simulink model "SimulinkProject"  (R2025b)
settings: Solver=ode5  StartTime=0.0  StopTime=60*5  FixedStep=1/16000  RelTol=1e-3
model workspace (MAT data in the model file):
  mass = 7
  radius = 333
undefined symbols (not defined in the file): DiscIntNeverNeededParam
libraries: simulink x5, simulink_extras x4, eeGeneralControl x2
settings Model: Creator=Fabian  LastModifiedBy=Fabian

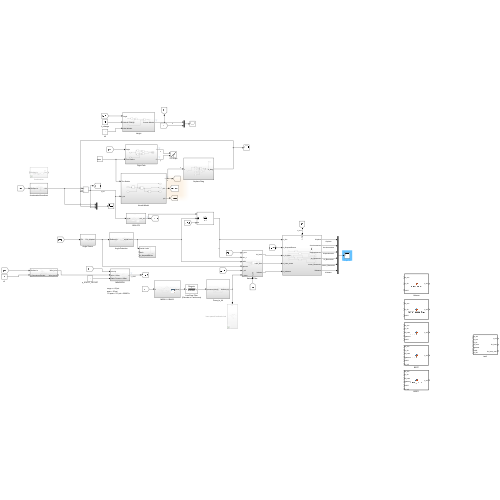
[thumbnail: Simulink's stored preview of the top-level diagram]
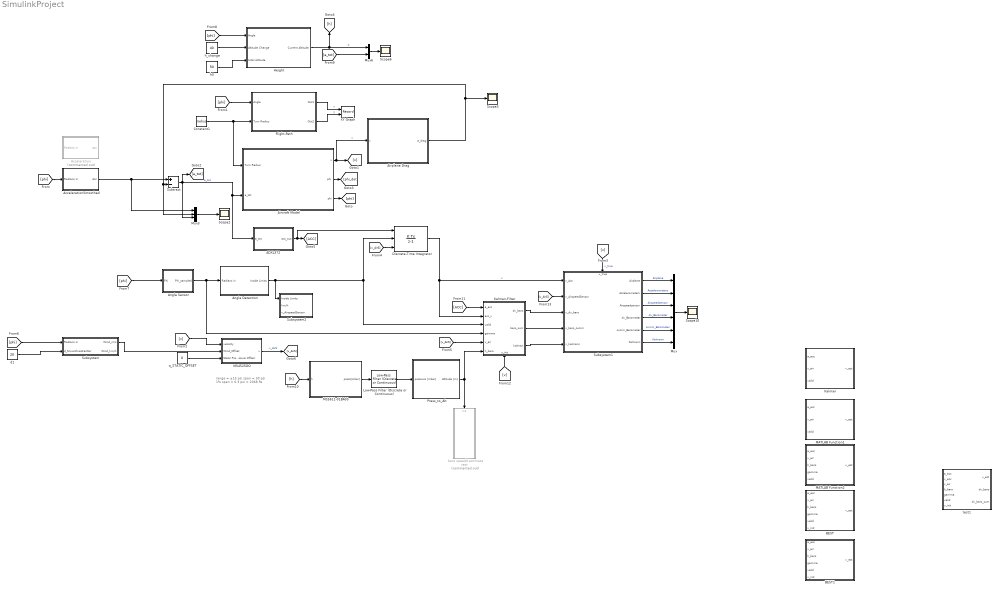
== system SimulinkProject ==
  note: range = ±15 psi
      | span = 30 psi
      | 1% span = 0.3 psi ≈ 2068 Pa
  ADXL372 : Subsystem
  Acceleration : Subsystem  Commented=on
  AccelerationSmoothed : Subsystem
  Aircraft Model : Subsystem
  Airplane Drag : Subsystem
  Angle Detection : Subsystem
  Angle Sensor : Subsystem
  BEST : MATLAB Function  TreatAsAtomicUnit=on
  BEST1 : MATLAB Function  TreatAsAtomicUnit=on
  Constant1 : Constant  Value=radius
  Discrete-Time Integrator : DiscreteIntegrator  ExternalReset=level  InitialConditionSource=external  SampleTime=1/3200  ICPrevOutput=DiscIntNeverNeededParam  ICPrevScaledInput=DiscIntNeverNeededParam
  Flight-Path : Subsystem
  Height : Subsystem
  Kalman : MATLAB Function  TreatAsAtomicUnit=on
  Kalman-Filter : Subsystem
      settings: PortSchema="{\"entries\":[{\"content\":{\"sides\":[{\"content\":{\"connectorIds\":[\"In1\",\"In2\",\"In3\",\"In4\",\"In5\",\"In6\"]},\"type\":\"ConnectorPlacement.EquallySpacedRectSide\",\"uuid\":\"52a043f1-34d7-4573-920f-90bbef37c175\"},{\"content\":{\"connectorIds\":[\"Out1\",\"Out2\",\"Out3\"],\"side\":\"RIGHT\"},\"type\":\"ConnectorPlacement.EquallySpacedRectSide\",\"uuid\":\"45beeb02-59fe-4ad5-aebe-ddb1f1721e27\"},{\"content\":{\"side\":\"TOP\"},\"type\":\"ConnectorPlacement.EquallySpacedRectSide\",\"uuid\":\"02723afe-8ee2-4376-9f83-f239e2e6ab52\"},{\"content\":{\"connectorIds\":[\"In7\"],\"side\":\"BOTTOM\"},\"type\":\"ConnectorPlacement.EquallySpacedRectSide\",\"uuid\":\"f847a05c-6e0c-45de-94de-b2ed33ea680b\"}]},\"type\":\"ConnectorPlacement.EquallySpacedConnector\",\"uuid\":\"0a8bc44f-e3ea-43fc-9907-5bdc9879c4d9\"}],\"packageUris\":[\"http://schema.mathworks.com/mf0/Connector/R2020b\"],\"version\":\"1.0\"}"
  Low-Pass Filter (Discrete or Continuous) : eeGeneralControl/Low-Pass Filter (Discrete or Continuous)  K=1  T=0.021  B=inf  A=-inf  init_option=Inherited from block input  x0=0  Ts=-1
  MATLAB Function1 : MATLAB Function  TreatAsAtomicUnit=on
  MATLAB Function2 : MATLAB Function  TreatAsAtomicUnit=on
  MS4525DO : Subsystem
  "MS5611-01BA03 " : Subsystem
  Mux : Mux  Inputs=6
  Mux3 : Mux  Inputs=3
  Mux6 : Mux  Inputs=2
  Press_to_Alt : Subsystem
  Scope{2..3,6,10} (4 alike) : Scope
      Scope10 settings: ActiveDisplayYMinimum=748.19267918173944  ActiveDisplayYMaximum=894.80486408784191  DataLoggingVariableName=ScopeData11
      Scope2 settings: ActiveDisplayYMinimum=-39.208466924616559  ActiveDisplayYMaximum=63.33696033694325  DataLoggingVariableName=ScopeData3
      Scope3 settings: ActiveDisplayYMinimum=-3.5843354434410593  ActiveDisplayYMaximum=33.486381490969542  DataLoggingVariableName=ScopeData6
      Scope6 settings: ActiveDisplayYMinimum=-31.394100237137991  ActiveDisplayYMaximum=92.400581276019  DataLoggingVariableName=ScopeData13
  Subsystem : Subsystem
  Subsystem1 : Subsystem
      settings: PortSchema="{\"entries\":[{\"content\":{\"sides\":[{\"content\":{\"connectorIds\":[\"In1\",\"In2\",\"In3\",\"In4\",\"In5\"]},\"type\":\"ConnectorPlacement.EquallySpacedRectSide\",\"uuid\":\"1310de41-fa36-4b52-bea7-0cc5965a0e40\"},{\"content\":{\"connectorIds\":[\"Out1\",\"Out2\",\"Out3\",\"Out4\",\"Out5\",\"Out6\"],\"side\":\"RIGHT\"},\"type\":\"ConnectorPlacement.EquallySpacedRectSide\",\"uuid\":\"190a2e70-065a-4914-8f4e-4e8426a30cbe\"},{\"content\":{\"connectorIds\":[\"In6\"],\"side\":\"TOP\"},\"type\":\"ConnectorPlacement.EquallySpacedRectSide\",\"uuid\":\"6c2c139e-493e-4709-bc4f-803947cf8aa6\"}]},\"type\":\"ConnectorPlacement.EquallySpacedConnector\",\"uuid\":\"13196e14-1744-4a93-b58c-eb55a0754985\"}],\"packageUris\":[\"http://schema.mathworks.com/mf0/Connector/R2020b\"],\"version\":\"1.0\"}"
  Subsystem2 : Subsystem
  Subtract : Sum  Inputs=+-
  XY Graph : Record  NumPorts=2.0  FileSettingsInternal="{\"entries\":[{\"content\":{\"excelSettings\":{\"content\":{},\"type\":\"Streamout.ExcelSettings\"},\"parquetSettings\":{\"content\":{},\"type\":\"Streamout.ParquetSettings\"}},\"type\":\"Streamout.FileSettingStorage\",\"uuid\":\"\"}],\"packageUris\":[\"http:\\/\\/schema.mathworks.com\\/mf0\\/streamout_blocks\\/R2020a\"],\"version\":\"1.0\"}"  FrameSettings=[0, 0]  Layout=[1 1]  SignalsInternal="{\"entries\":[{\"content\":{\"signals\":[{\"content\":{\"blockPath\":[],\"dimensions\":[1],\"domain\":\"\",\"lineColor\":\"#a2142f\",\"plots\":[ 1 ],\"port\":1,\"sid\":[\"\"],\"signalID\":1,\"signalName\":\"x\"},\"type\":\"RecordBlkView.Signal\",\"uuid\":\"\"},{\"content\":{\"blockPath\":[],\"dimensions\":[1],\"domain\":\"\",\"lineColor\":\"#139fff\",\"plots\":[ 1 ],\"port\":2,\"sid\":[\"\"],\"signalID\":2,\"signalName\":\"y\"},\"type\":\"RecordBlkView.Signal\",\"uuid\":\"\"}]},\"type\":\"RecordBlkView.InputSignals\",\"uuid\":\"\"}],\"packageUris\":[\"http:\\/\\/schema.mathworks.com\\/mf0\\/streamout_blocks\\/R2020a\"],\"version\":\"1.0\"}"  VisualizationBindings="{\"xyplotplugin\":{\"info\":[{\"series\":[{\"bindingParametersList\":[{\"parameter\":\"X-Axis\",\"signalID\":1,\"signalName\":\"x\"},{\"parameter\":\"Y-Axis\",\"signalID\":2,\"signalName\":\"y\"}],\"seriesID\":0}],\"subplotID\":1}]}}"  CompatibilityTag=XY
  baro speedd estimate test : Subsystem  Commented=on
  d1 : Constant  Value=20
  h0 : Constant  Value=50
  h_change : Constant  Value=40
  q_STATIC_OFFSET : Constant  Value=0
  test1 : MATLAB Function  TreatAsAtomicUnit=on
  wires:
  Subtract/1 -> [a_tot], ADXL372/1(a_tot), Aircraft Model/2(a_tot), Mux3/3  "a_tot"
  Constant1/1 -> Flight-Path/2(Turn Radius), Aircraft Model/1(Turn Radius)
  [phi] -> AccelerationSmoothed/1(Radians in)
  [v] -> MS4525DO/1(velocity)
  q_STATIC_OFFSET/1 -> MS4525DO/3(Static Pressure Offset)
  [phi] -> Flight-Path/1(Angle)
  Flight-Path/1(Out1) -> XY Graph/1  "x"
  Flight-Path/2(Out2) -> XY Graph/2  "y"
  Aircraft Model/1(v) -> Airplane Drag/1(v), [v]  "v"
  Aircraft Model/2(phi.) -> [phi_dot]
  Aircraft Model/3(phi) -> [phi]
  Mux3/1 -> Scope2/1
  [phi] -> Subsystem/1(Radians in)
  d1/1 -> Subsystem/2(d_SmoothnesFacttor)
  Subsystem/1(Wind_m/s) -> MS4525DO/2(Wind_Offset)
  AccelerationSmoothed/1(Acc) -> Mux3/1, Subtract/1
  [phi] -> Angle Sensor/1(Phi)
  h0/1 -> Height/3(Inital altitude)
  h_change/1 -> Height/2(Altitude Change)
  [phi] -> Height/1(Angle)
  Mux6/1 -> Scope6/1
  Height/1(Current Altitude) -> [h], Mux6/1  "h"
  [a_tot] -> Mux6/2
  [h] -> "MS5611-01BA03 "/1(h)
  Airplane Drag/1(a_drag) -> Mux3/2, Subtract/2, Scope3/1
  Discrete-Time Integrator/1 -> Kalman-Filter/2(acc_v), Subsystem1/1(v_Acc)  "v"
  "MS5611-01BA03 "/1(press[mbar]) -> Low-Pass Filter (Discrete or Continuous)/1
  Press_to_Alt/1(Altitude [m]) -> Kalman-Filter/6(h_baro), baro speedd estimate test/1(In1)
  Low-Pass Filter (Discrete or Continuous)/1 -> Press_to_Alt/1(pressure [mbar])
  Angle Sensor/1(Phi_sampled) -> Kalman-Filter/4(gamma), Angle Detection/1(Radians in)
  Angle Detection/1(Inside Limits) -> Subsystem2/1(Inside Limits), Kalman-Filter/3(valid), Discrete-Time Integrator/2
  ADXL372/1(acc_out) -> Discrete-Time Integrator/1, [ACC]
  [ACC] -> Kalman-Filter/1(a_acc)
  [v] -> Kalman-Filter/7(v_init)
  MS4525DO/1(v) -> [v_AirS]  "v_AirS"
  [v_AirS] -> Discrete-Time Integrator/3
  [v_AirS] -> Kalman-Filter/5(v_air)
  [v] -> Subsystem1/6(v_true)  "v_true"
  [v_AirS] -> Subsystem1/2(v_AirspeedSensor)
  Kalman-Filter/1(dv_baro) -> Subsystem1/3(v_dv_baro)
  Kalman-Filter/2(baro_sum) -> Subsystem1/4(v_baro_summ)
  Kalman-Filter/3(kalman) -> Subsystem1/5(v_kalmann)
  Mux/1 -> Scope10/1
  Subsystem1/1(Airplane) -> Mux/1  "Airplane"
  Subsystem1/2(Accelerometers) -> Mux/2  "Accelerometers"
  Subsystem1/3(Airspeedsensor) -> Mux/3  "Airspeedsensor"
  Subsystem1/4(dv_Barometer) -> Mux/4  "dv_Barometer"
  Subsystem1/5(summ_Barometer) -> Mux/5  "summ_Barometer"
  Subsystem1/6(Kalmann) -> Mux/6  "Kalmann"

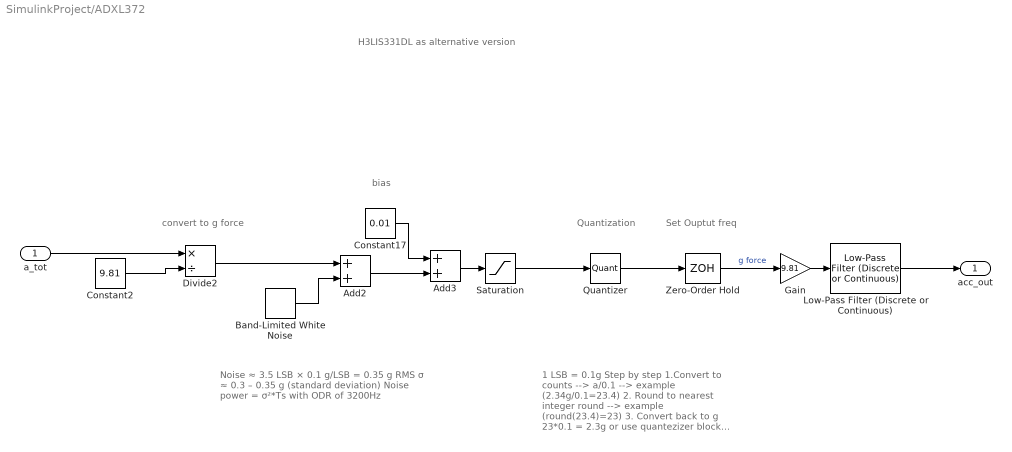
== system SimulinkProject/ADXL372 ==
  note: H3LIS331DL as alternative version
  note: convert to g force
  note: Noise ≈ 3.5 LSB × 0.1 g/LSB = 0.35 g RMS
      | σ ≈ 0.3 – 0.35 g (standard deviation)
      | Noise power = σ²*Ts
      | with ODR of 3200Hz
  note: bias
  note: Quantization
  note: 1 LSB = 0.1g
      | Step by step
      |
      | 1.Convert to counts
      | --> a/0.1 --> example (2.34g/0.1=23.4)
      | 2. Round to nearest integer
      | round --> example (round(23.4)=23)
      | 3. Convert back to g
      | 23*0.1 = 2.3g
      |
      | or use quantezizer block with 0.1
  note: Set Ouptut freq
  a_tot : Inport
  Add2 : Sum
  Add3 : Sum
  Band-Limited White Noise : simulink/Sources/Band-Limited White Noise  Cov=((0.35)^2)*(1/3200)  Ts=1/3200  seed=[23341]
  Constant17 : Constant  Value=0.01
  Constant2 : Constant  Value=9.81
  Divide2 : Product  Inputs=*/
  Gain : Gain  Gain=9.81
  Low-Pass Filter (Discrete or Continuous) : eeGeneralControl/Low-Pass Filter (Discrete or Continuous)  K=1  T=1/(2*pi*10)  B=inf  A=-inf  init_option=Inherited from block input  x0=0  Ts=1/3200
  Quantizer : Quantizer  QuantizationInterval=0.1
  Saturation : Saturate  UpperLimit=200  LowerLimit=-200
  Zero-Order Hold : ZeroOrderHold  SampleTime=1/3200
  acc_out : Outport
  wires:
  Constant2/1 -> Divide2/2
  Add3/1 -> Saturation/1
  Saturation/1 -> Quantizer/1
  Divide2/1 -> Add2/1
  Gain/1 -> Low-Pass Filter (Discrete or Continuous)/1
  Add2/1 -> Add3/2
  Constant17/1 -> Add3/1
  Band-Limited White Noise/1 -> Add2/2
  Quantizer/1 -> Zero-Order Hold/1
  Zero-Order Hold/1 -> Gain/1  "g force"
  Low-Pass Filter (Discrete or Continuous)/1 -> acc_out/1
  a_tot/1 -> Divide2/1

== system SimulinkProject/Acceleration ==
  note: Case 0 --> (0>value<120)
      | Case 1 --> (120>value<200)
      | Case 2 --> (200>value <360)
  Radians in : Inport
  1-D Lookup Table : Lookup_n-D  NumberOfTableDimensions=1  BreakpointsForDimension1=[0 120 130 190 210 360]  Table=[-3 -3 6 6 4 4]  InterpMethod=Linear Lagrange  InternalRulePriority=Speed  RndMeth=Simplest
  Constant4 : Constant  Value=360
  Math Function : Math  Operator=mod
  Radians to Degrees : simulink_extras/Transformations/Radians to Degrees
  Scope1 : Scope
      settings: ActiveDisplayYMinimum=2.9529948597935629  ActiveDisplayYMaximum=755.41634315848091
  Acc : Outport
  wires:
  Radians to Degrees/1 -> Math Function/1
  Constant4/1 -> Math Function/2
  Math Function/1 -> Scope1/1, 1-D Lookup Table/1
  Radians in/1 -> Radians to Degrees/1
  1-D Lookup Table/1 -> Acc/1

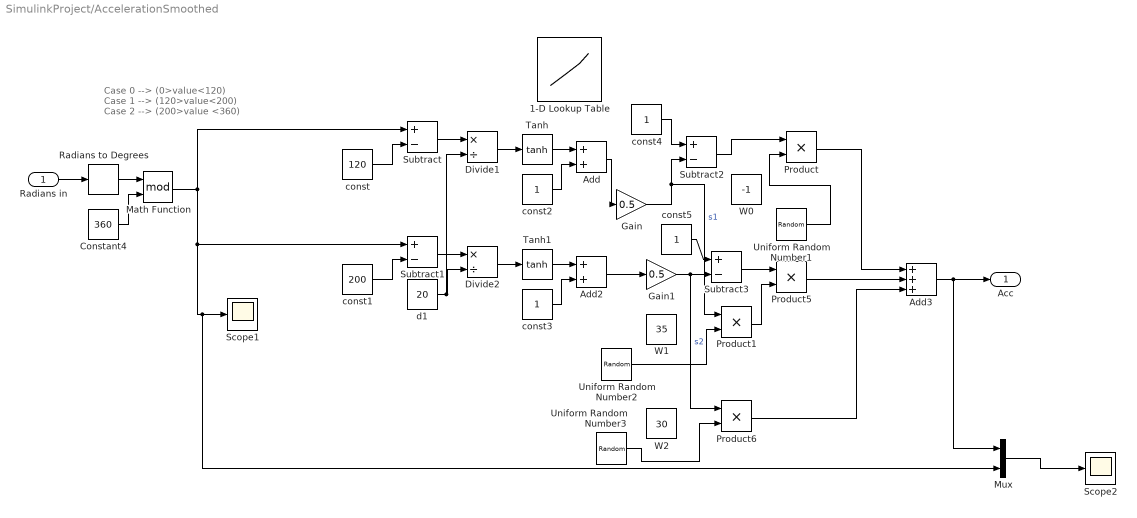
== system SimulinkProject/AccelerationSmoothed ==
  note: Case 0 --> (0>value<120)
      | Case 1 --> (120>value<200)
      | Case 2 --> (200>value <360)
  Radians in : Inport
  1-D Lookup Table : Lookup_n-D  NumberOfTableDimensions=1  BreakpointsForDimension1=[0 110 130 190 210 360]  Table=[-3 -3 6 6 4 4]  InterpMethod=Linear Lagrange  InternalRulePriority=Speed  RndMeth=Simplest
  Add : Sum
  Add2 : Sum
  Add3 : Sum  Inputs=+++
  Constant4 : Constant  Value=360
  Divide1 : Product  Inputs=*/
  Divide2 : Product  Inputs=*/
  Gain : Gain  Gain=0.5
  Gain1 : Gain  Gain=0.5
  Math Function : Math  Operator=mod
  Mux : Mux  Inputs=2
  Product{,1,5..6} (4 alike) : Product
  Radians to Degrees : simulink_extras/Transformations/Radians to Degrees
  Scope1 : Scope
      settings: ActiveDisplayYMinimum=-47.332509505790171  ActiveDisplayYMaximum=913.02258838484045
  Scope2 : Scope
      settings: ActiveDisplayYMinimum=-16.733117928341755  ActiveDisplayYMaximum=372.27391286785394  DataLoggingVariableName=ScopeData5
  Subtract{,1..3} (4 alike) : Sum  Inputs=+-
  Tanh : Trigonometry  Operator=tanh
  Tanh1 : Trigonometry  Operator=tanh
  Uniform Random Number1 : UniformRandomNumber  Minimum=-2  Maximum=0  SampleTime=0.1
  Uniform Random Number2 : UniformRandomNumber  Minimum=30  Maximum=40  SampleTime=0.1
  Uniform Random Number3 : UniformRandomNumber  Minimum=25  Maximum=35  SampleTime=0.1
  W0 : Constant  Value=-1
  W1 : Constant  Value=35
  W2 : Constant  Value=30
  const : Constant  Value=120
  const1 : Constant  Value=200
  const{2..5} (4 alike) : Constant
  d1 : Constant  Value=20
  Acc : Outport
  wires:
  Radians to Degrees/1 -> Math Function/1
  Constant4/1 -> Math Function/2
  Radians in/1 -> Radians to Degrees/1
  Math Function/1 -> Subtract1/1, Mux/2, Scope1/1, Subtract/1
  const4/1 -> Subtract2/1
  Tanh/1 -> Add/1
  const2/1 -> Add/2
  Add/1 -> Gain/1
  Product1/1 -> Product5/2
  Tanh1/1 -> Add2/1
  Subtract3/1 -> Product5/1
  Product6/1 -> Add3/3
  Subtract2/1 -> Product/1
  Subtract/1 -> Divide1/1
  const3/1 -> Add2/2
  Divide1/1 -> Tanh/1
  const/1 -> Subtract/2
  const1/1 -> Subtract1/2
  Subtract1/1 -> Divide2/1
  d1/1 -> Divide1/2, Divide2/2
  const5/1 -> Subtract3/1
  Gain1/1 -> Product6/1, Subtract3/2  "s2"
  Product5/1 -> Add3/2
  Add2/1 -> Gain1/1
  Gain/1 -> Subtract2/2, Product1/1  "s1"
  Divide2/1 -> Tanh1/1
  Product/1 -> Add3/1
  Add3/1 -> Mux/1, Acc/1
  Mux/1 -> Scope2/1
  Uniform Random Number1/1 -> Product/2
  Uniform Random Number2/1 -> Product1/2
  Uniform Random Number3/1 -> Product6/2

== system SimulinkProject/Aircraft Model ==
  Turn Radius : Inport
  a_tot : Inport  Port=2
  Divide1 : Product  Inputs=*/
  Integrator2 : Integrator  InitialCondition=13
  Integrator3 : Integrator  InitialCondition=pi
  v : Outport
  phi. : Outport  Port=2
  phi : Outport  Port=3
  wires:
  Divide1/1 -> phi./1, Integrator3/1  "phi."
  Integrator3/1 -> phi/1
  Integrator2/1 -> v/1, Divide1/1  "v"
  Turn Radius/1 -> Divide1/2
  a_tot/1 -> Integrator2/1

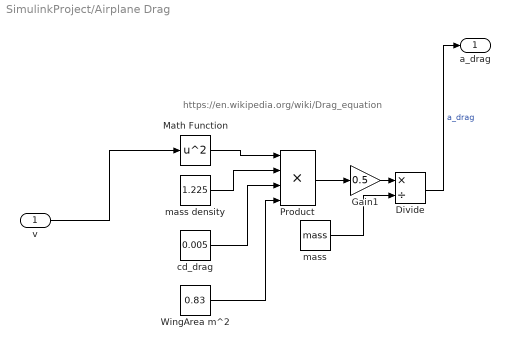
== system SimulinkProject/Airplane Drag ==
  note: https://en.wikipedia.org/wiki/Drag_equation
  v : Inport
  Divide : Product  Inputs=*/
  Gain1 : Gain  Gain=0.5
  Math Function : Math  Operator=square
  Product : Product  Inputs=4
  WingArea m^2 : Constant  Value=0.83
  cd_drag : Constant  Value=0.005
  mass : Constant  Value=mass
  mass density : Constant  Value=1.225
  a_drag : Outport
  wires:
  mass/1 -> Divide/2
  mass density/1 -> Product/2
  Divide/1 -> a_drag/1  "a_drag"
  Math Function/1 -> Product/1
  cd_drag/1 -> Product/3
  Gain1/1 -> Divide/1
  WingArea m^2/1 -> Product/4
  Product/1 -> Gain1/1
  v/1 -> Math Function/1

== system SimulinkProject/Angle Detection ==
  Radians in : Inport
  Compare To Constant : simulink/Logic and Bit Operations/Compare To Constant  relop=>=  const=50  OutDataTypeStr=boolean
  Compare To Constant1 : simulink/Logic and Bit Operations/Compare To Constant  relop=<=  const=80  OutDataTypeStr=boolean
  Constant4 : Constant  Value=360
  Logical Operator : Logic  AllPortsSameDT=off  OutDataTypeStr=fixdt(1,16)
  Math Function1 : Math  Operator=mod
  Radians to Degrees : simulink_extras/Transformations/Radians to Degrees
  Inside Limits : Outport
  wires:
  Math Function1/1 -> Compare To Constant/1, Compare To Constant1/1
  Compare To Constant/1 -> Logical Operator/1
  Compare To Constant1/1 -> Logical Operator/2
  Radians to Degrees/1 -> Math Function1/1
  Constant4/1 -> Math Function1/2
  Logical Operator/1 -> Inside Limits/1
  Radians in/1 -> Radians to Degrees/1

== system SimulinkProject/Angle Sensor ==
  Phi : Inport
  Zero-Order Hold3 : ZeroOrderHold  SampleTime=1/3200
  Phi_sampled : Outport
  wires:
  Zero-Order Hold3/1 -> Phi_sampled/1
  Phi/1 -> Zero-Order Hold3/1

== system SimulinkProject/Flight-Path ==
  Angle : Inport
  Turn Radius : Inport  Port=2
  Cos : Trigonometry  Operator=cos
  Cos1 : Trigonometry
  Product : Product
  Product1 : Product
  Out1 : Outport
  Out2 : Outport  Port=2
  wires:
  Cos1/1 -> Product1/2
  Turn Radius/1 -> Product/2, Product1/1
  Angle/1 -> Cos1/1, Cos/1
  Cos/1 -> Product/1
  Product1/1 -> Out2/1
  Product/1 -> Out1/1

== system SimulinkProject/Height ==
  Angle : Inport
  Altitude Change : Inport  Port=2
  Inital altitude : Inport  Port=3
  Add : Sum
  Cos1 : Trigonometry
  Product : Product
  Current Altitude : Outport
  wires:
  Angle/1 -> Cos1/1
  Inital altitude/1 -> Add/2
  Altitude Change/1 -> Product/2
  Cos1/1 -> Product/1
  Product/1 -> Add/1
  Add/1 -> Current Altitude/1

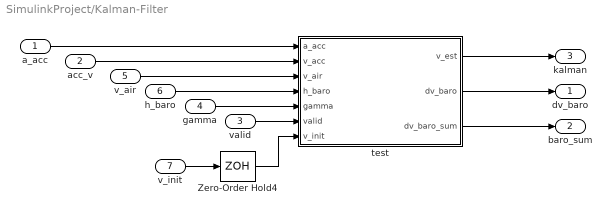
== system SimulinkProject/Kalman-Filter ==
  a_acc : Inport
  acc_v : Inport  Port=2
  valid : Inport  Port=3
  gamma : Inport  Port=4
  v_air : Inport  Port=5
  h_baro : Inport  Port=6
  v_init : Inport  Port=7
  Zero-Order Hold4 : ZeroOrderHold  SampleTime=1/3200
  test : MATLAB Function  TreatAsAtomicUnit=on
  dv_baro : Outport
  baro_sum : Outport  Port=2
  kalman : Outport  Port=3
  wires:
  v_init/1 -> Zero-Order Hold4/1
  acc_v/1 -> test/2(v_acc)
  Zero-Order Hold4/1 -> test/7(v_init)
  h_baro/1 -> test/4(h_baro)
  valid/1 -> test/6(valid)
  v_air/1 -> test/3(v_air)
  gamma/1 -> test/5(gamma)
  test/1(v_est) -> kalman/1
  test/2(dv_baro) -> dv_baro/1
  test/3(dv_baro_sum) -> baro_sum/1
  a_acc/1 -> test/1(a_acc)

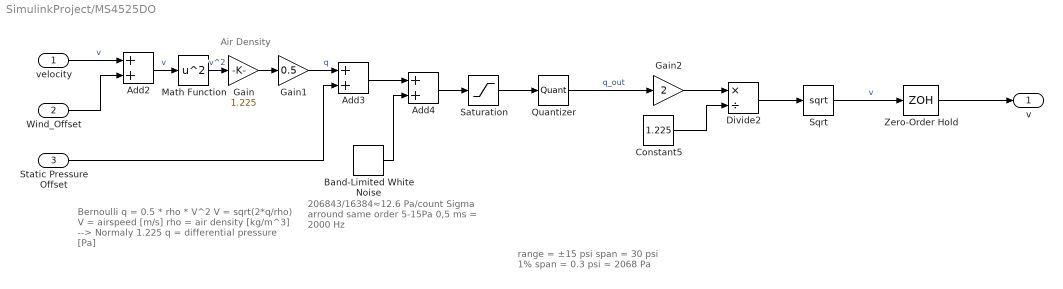
== system SimulinkProject/MS4525DO ==
  note: Bernoulli
      | q = 0.5 * rho * V^2
      | V = sqrt(2*q/rho)
      |
      | V = airspeed [m/s]
      | rho = air density [kg/m^3] --> Normaly 1.225
      | q = differential pressure [Pa]
  note: Air Density
  note: 206843/16384​≈12.6 Pa/count
      | Sigma arround same order 5-15Pa
      |
      | 0,5 ms = 2000 Hz
  note: range = ±15 psi
      | span = 30 psi
      | 1% span = 0.3 psi ≈ 2068 Pa
  velocity : Inport
  Wind_Offset : Inport  Port=2
  Static Pressure Offset : Inport  Port=3
  Add2 : Sum
  Add3 : Sum
  Add4 : Sum
  Band-Limited White Noise : simulink/Sources/Band-Limited White Noise  Cov=((10)^2)*(1/2000)  Ts=1/2000  seed=[23341]
  Constant5 : Constant  Value=1.225
  Divide2 : Product  Inputs=*/
  Gain : Gain  Gain=1.225
  Gain1 : Gain  Gain=0.5
  Gain2 : Gain  Gain=2
  Math Function : Math  Operator=square
  Quantizer : Quantizer  QuantizationInterval=12.6
  Saturation : Saturate  UpperLimit=103421  LowerLimit=-103421
  Sqrt : Sqrt
  Zero-Order Hold : ZeroOrderHold  SampleTime=1/2000
  v : Outport
  wires:
  Add3/1 -> Add4/1
  Divide2/1 -> Sqrt/1
  Add2/1 -> Math Function/1  "v"
  Saturation/1 -> Quantizer/1
  Math Function/1 -> Gain/1  "v^2"
  Gain/1 -> Gain1/1
  Gain1/1 -> Add3/1  "q"
  Add4/1 -> Saturation/1
  Gain2/1 -> Divide2/1
  Wind_Offset/1 -> Add2/2
  Constant5/1 -> Divide2/2
  Quantizer/1 -> Gain2/1  "q_out"
  Band-Limited White Noise/1 -> Add4/2
  velocity/1 -> Add2/1  "v"
  Static Pressure Offset/1 -> Add3/2
  Sqrt/1 -> Zero-Order Hold/1  "v"
  Zero-Order Hold/1 -> v/1

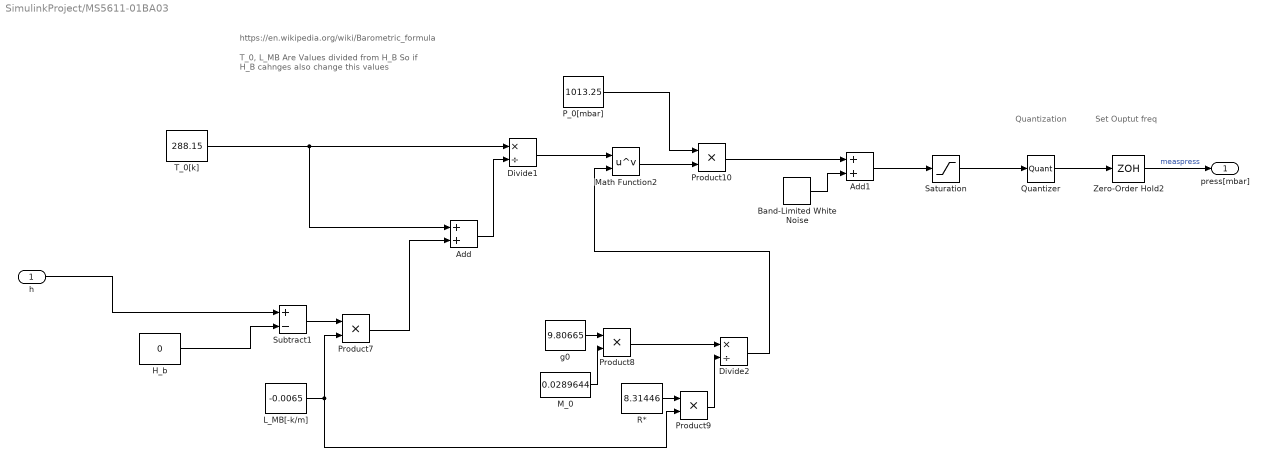
== system SimulinkProject/MS5611-01BA03  ==
  note: https://en.wikipedia.org/wiki/Barometric_formula
  note: T_0, L_MB
      | Are Values divided from H_B
      | So if H_B cahnges also change this values
  note: Set Ouptut freq
  note: Quantization
  h : Inport
  Add : Sum
  Add1 : Sum
  Band-Limited White Noise : simulink/Sources/Band-Limited White Noise  Cov=(0.065)^2 * (1/2000)  Ts=1/2000  seed=[23341]
  Divide1 : Product  Inputs=*/
  Divide2 : Product  Inputs=*/
  H_b : Constant  Value=0
  L_MB[-k/m] : Constant  Value=-0.0065
  M_0 : Constant  Value=0.0289644
  Math Function2 : Math  Operator=pow
  P_0[mbar] : Constant  Value=1013.25
  Product{7..10} (4 alike) : Product
  Quantizer : Quantizer  QuantizationInterval=(1200-10)/(2^24)
  R* : Constant  Value=8.31446
  Saturation : Saturate  UpperLimit=1200  LowerLimit=10
  Subtract1 : Sum  Inputs=+-
  T_0[k] : Constant  Value=288.15
  Zero-Order Hold2 : ZeroOrderHold  SampleTime=1/2000
  g0 : Constant  Value=9.80665
  press[mbar] : Outport
  wires:
  R*/1 -> Product9/1
  L_MB[-k/m]/1 -> Product9/2, Product7/2
  Product9/1 -> Divide2/2
  g0/1 -> Product8/1
  h/1 -> Subtract1/1
  M_0/1 -> Product8/2
  T_0[k]/1 -> Add/1, Divide1/1
  Add/1 -> Divide1/2
  Subtract1/1 -> Product7/1
  P_0[mbar]/1 -> Product10/1
  Math Function2/1 -> Product10/2
  Product7/1 -> Add/2
  Divide2/1 -> Math Function2/2
  H_b/1 -> Subtract1/2
  Product8/1 -> Divide2/1
  Divide1/1 -> Math Function2/1
  Quantizer/1 -> Zero-Order Hold2/1
  Band-Limited White Noise/1 -> Add1/2
  Add1/1 -> Saturation/1
  Zero-Order Hold2/1 -> press[mbar]/1  "measpress"
  Saturation/1 -> Quantizer/1
  Product10/1 -> Add1/1

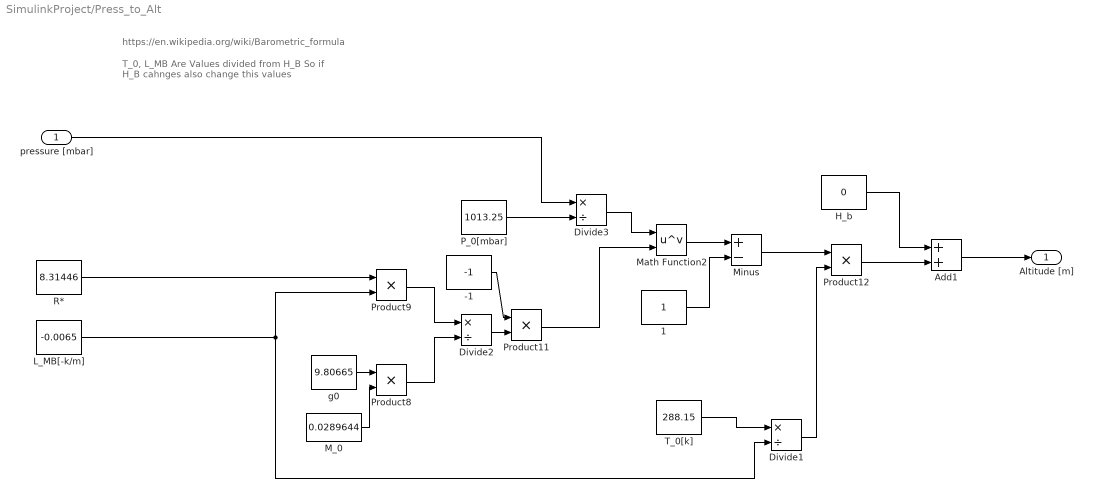
== system SimulinkProject/Press_to_Alt ==
  note: https://en.wikipedia.org/wiki/Barometric_formula
  note: T_0, L_MB
      | Are Values divided from H_B
      | So if H_B cahnges also change this values
  pressure [mbar] : Inport
  -1 : Constant  Value=-1
  1 : Constant
  Add1 : Sum
  Divide1 : Product  Inputs=*/
  Divide2 : Product  Inputs=*/
  Divide3 : Product  Inputs=*/
  H_b : Constant  Value=0
  L_MB[-k/m] : Constant  Value=-0.0065
  M_0 : Constant  Value=0.0289644
  Math Function2 : Math  Operator=pow
  Minus : Sum  Inputs=+-
  P_0[mbar] : Constant  Value=1013.25
  Product{8..9,11..12} (4 alike) : Product
  R* : Constant  Value=8.31446
  T_0[k] : Constant  Value=288.15
  g0 : Constant  Value=9.80665
  Altitude [m] : Outport
  wires:
  Product12/1 -> Add1/2
  Product11/1 -> Math Function2/2
  Product8/1 -> Divide2/2
  g0/1 -> Product8/1
  1/1 -> Minus/2
  Product9/1 -> Divide2/1
  -1/1 -> Product11/1
  L_MB[-k/m]/1 -> Product9/2, Divide1/2
  M_0/1 -> Product8/2
  Math Function2/1 -> Minus/1
  Divide3/1 -> Math Function2/1
  H_b/1 -> Add1/1
  R*/1 -> Product9/1
  Divide1/1 -> Product12/2
  Minus/1 -> Product12/1
  T_0[k]/1 -> Divide1/1
  Divide2/1 -> Product11/2
  P_0[mbar]/1 -> Divide3/2
  pressure [mbar]/1 -> Divide3/1
  Add1/1 -> Altitude [m]/1

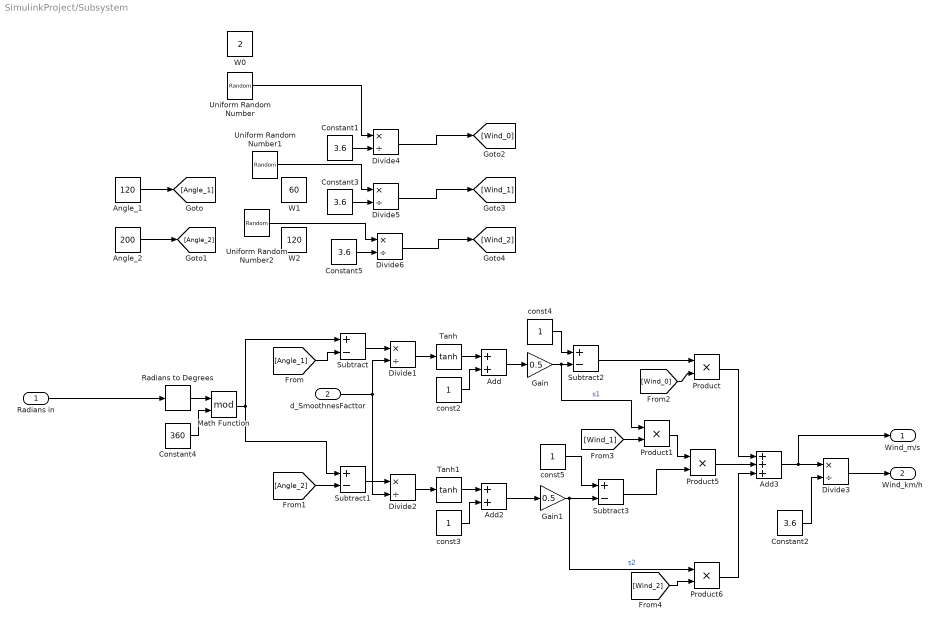
== system SimulinkProject/Subsystem ==
  Radians in : Inport
  d_SmoothnesFacttor : Inport  Port=2
  Add : Sum
  Add2 : Sum
  Add3 : Sum  Inputs=+++
  Angle_1 : Constant  Value=120
  Angle_2 : Constant  Value=200
  Constant{1..3,5} (4 alike) : Constant  Value=3.6
  Constant4 : Constant  Value=360
  Divide{1..6} (6 alike) : Product  Inputs=*/
  Gain : Gain  Gain=0.5
  Gain1 : Gain  Gain=0.5
  Math Function : Math  Operator=mod
  Product{,1,5..6} (4 alike) : Product
  Radians to Degrees : simulink_extras/Transformations/Radians to Degrees
  Subtract{,1..3} (4 alike) : Sum  Inputs=+-
  Tanh : Trigonometry  Operator=tanh
  Tanh1 : Trigonometry  Operator=tanh
  Uniform Random Number : UniformRandomNumber  Minimum=0  Maximum=10  SampleTime=0.1
  Uniform Random Number1 : UniformRandomNumber  Minimum=50  Maximum=70  SampleTime=0.1
  Uniform Random Number2 : UniformRandomNumber  Minimum=110  Maximum=130  SampleTime=0.1
  W0 : Constant  Value=2
  W1 : Constant  Value=60
  W2 : Constant  Value=120
  const{2..5} (4 alike) : Constant
  Wind_m/s : Outport
  Wind_km/h : Outport  Port=2
  wires:
  Math Function/1 -> Subtract/1, Subtract1/1
  Divide3/1 -> Wind_km/h/1
  Subtract1/1 -> Divide2/1
  Gain/1 -> Product1/1, Subtract2/2  "s1"
  Divide2/1 -> Tanh1/1
  Gain1/1 -> Subtract3/2, Product6/1  "s2"
  Product6/1 -> Add3/3
  Subtract2/1 -> Product/1
  Divide1/1 -> Tanh/1
  const2/1 -> Add/2
  Constant2/1 -> Divide3/2
  Subtract/1 -> Divide1/1
  const3/1 -> Add2/2
  Tanh1/1 -> Add2/1
  Product/1 -> Add3/1
  Add/1 -> Gain/1
  Add3/1 -> Wind_m/s/1, Divide3/1
  Tanh/1 -> Add/1
  d_SmoothnesFacttor/1 -> Divide2/2, Divide1/2
  Radians to Degrees/1 -> Math Function/1
  const4/1 -> Subtract2/1
  const5/1 -> Subtract3/1
  Product5/1 -> Add3/2
  Constant4/1 -> Math Function/2
  Add2/1 -> Gain1/1
  Radians in/1 -> Radians to Degrees/1
  Angle_1/1 -> [Angle_1]
  [Angle_1] -> Subtract/2
  Angle_2/1 -> [Angle_2]
  [Angle_2] -> Subtract1/2
  [Wind_0] -> Product/2
  [Wind_1] -> Product1/2
  Subtract3/1 -> Product5/2
  Product1/1 -> Product5/1
  [Wind_2] -> Product6/2
  Constant1/1 -> Divide4/2
  Divide4/1 -> [Wind_0]
  Constant3/1 -> Divide5/2
  Divide5/1 -> [Wind_1]
  Constant5/1 -> Divide6/2
  Divide6/1 -> [Wind_2]
  Uniform Random Number/1 -> Divide4/1
  Uniform Random Number1/1 -> Divide5/1
  Uniform Random Number2/1 -> Divide6/1

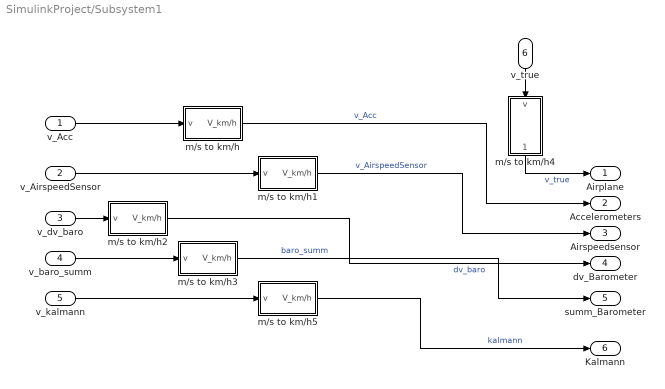
== system SimulinkProject/Subsystem1 ==
  v_Acc : Inport
  v_AirspeedSensor : Inport  Port=2
  v_dv_baro : Inport  Port=3
  v_baro_summ : Inport  Port=4
  v_kalmann : Inport  Port=5
  v_true : Inport  Port=6
  m/s to km/h : Subsystem
  m/s to km/h1 : Subsystem
  m/s to km/h2 : Subsystem
  m/s to km/h3 : Subsystem
  m/s to km/h4 : Subsystem
  m/s to km/h5 : Subsystem
  Airplane : Outport
  Accelerometers : Outport  Port=2
  Airspeedsensor : Outport  Port=3
  dv_Barometer : Outport  Port=4
  summ_Barometer : Outport  Port=5
  Kalmann : Outport  Port=6
  wires:
  v_true/1 -> m/s to km/h4/1(v)
  m/s to km/h4/1(V_km/h) -> Airplane/1  "v_true"
  m/s to km/h/1(V_km/h) -> Accelerometers/1  "v_Acc"
  m/s to km/h1/1(V_km/h) -> Airspeedsensor/1  "v_AirspeedSensor"
  v_Acc/1 -> m/s to km/h/1(v)
  v_AirspeedSensor/1 -> m/s to km/h1/1(v)
  v_dv_baro/1 -> m/s to km/h2/1(v)
  v_baro_summ/1 -> m/s to km/h3/1(v)
  v_kalmann/1 -> m/s to km/h5/1(v)
  m/s to km/h2/1(V_km/h) -> dv_Barometer/1  "dv_baro"
  m/s to km/h3/1(V_km/h) -> summ_Barometer/1  "baro_summ"
  m/s to km/h5/1(V_km/h) -> Kalmann/1  "kalmann"

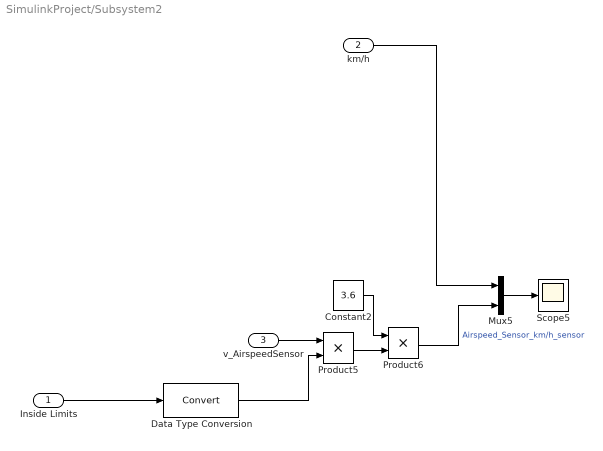
== system SimulinkProject/Subsystem2 ==
  Inside Limits : Inport
  km/h : Inport  Port=2
  v_AirspeedSensor : Inport  Port=3
  Constant2 : Constant  Value=3.6
  Data Type Conversion : DataTypeConversion  SaturateOnIntegerOverflow=off  RndMeth=Floor
  Mux5 : Mux  Inputs=2
  Product5 : Product
  Product6 : Product
  Scope5 : Scope
      settings: ActiveDisplayYMinimum=-118.47422406050404  ActiveDisplayYMaximum=1066.2680165445367  DataLoggingVariableName=ScopeData12
  wires:
  Mux5/1 -> Scope5/1
  v_AirspeedSensor/1 -> Product5/1
  Constant2/1 -> Product6/1
  Product5/1 -> Product6/2
  Inside Limits/1 -> Data Type Conversion/1
  Product6/1 -> Mux5/2  "Airspeed_Sensor_km/h_sensor"
  km/h/1 -> Mux5/1
  Data Type Conversion/1 -> Product5/2

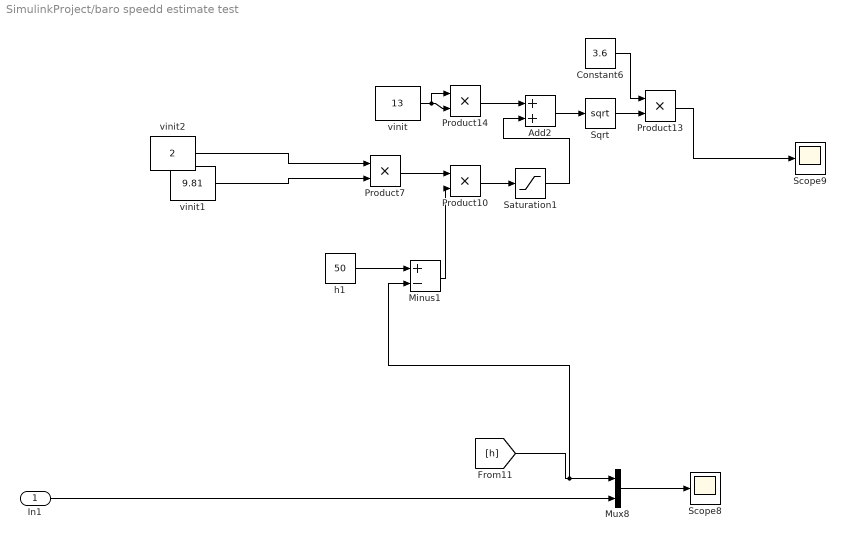
== system SimulinkProject/baro speedd estimate test ==
  In1 : Inport
  Add2 : Sum
  Constant6 : Constant  Value=3.6
  Minus1 : Sum  Inputs=+-
  Mux8 : Mux  Inputs=2
  Product{7,10,13..14} (4 alike) : Product
  Saturation1 : Saturate  UpperLimit=inf  LowerLimit=0.1
  Scope8 : Scope
      settings: ActiveDisplayYMinimum=85.0381751510035  ActiveDisplayYMaximum=91.4462483318631  DataLoggingVariableName=ScopeData15
  Scope9 : Scope
      settings: ActiveDisplayYMinimum=38.767930934422381  ActiveDisplayYMaximum=119.22706265224174  DataLoggingVariableName=ScopeData16
  Sqrt : Sqrt
  h1 : Constant  Value=50
  vinit : Constant  Value=13
  vinit1 : Constant  Value=9.81
  vinit2 : Constant  Value=2
  wires:
  Sqrt/1 -> Product13/2
  Minus1/1 -> Product10/2
  [h] -> Minus1/2, Mux8/1
  vinit1/1 -> Product7/2
  vinit2/1 -> Product7/1
  h1/1 -> Minus1/1
  Product14/1 -> Add2/1
  Product13/1 -> Scope9/1
  In1/1 -> Mux8/2
  Mux8/1 -> Scope8/1
  Product7/1 -> Product10/1
  Product10/1 -> Saturation1/1
  vinit/1 -> Product14/1, Product14/2
  Add2/1 -> Sqrt/1
  Saturation1/1 -> Add2/2
  Constant6/1 -> Product13/1

== system SimulinkProject/Subsystem1/m//s to km//h ==
  v : Inport
  Constant18 : Constant  Value=3.6
  Product3 : Product
  V_km/h : Outport
  wires:
  Constant18/1 -> Product3/1
  Product3/1 -> V_km/h/1
  v/1 -> Product3/2

== system SimulinkProject/Subsystem1/m//s to km//h1 ==
  v : Inport
  Constant18 : Constant  Value=3.6
  Product3 : Product
  V_km/h : Outport
  wires:
  Constant18/1 -> Product3/1
  Product3/1 -> V_km/h/1
  v/1 -> Product3/2

== system SimulinkProject/Subsystem1/m//s to km//h2 ==
  v : Inport
  Constant18 : Constant  Value=3.6
  Product3 : Product
  V_km/h : Outport
  wires:
  Constant18/1 -> Product3/1
  Product3/1 -> V_km/h/1
  v/1 -> Product3/2

== system SimulinkProject/Subsystem1/m//s to km//h3 ==
  v : Inport
  Constant18 : Constant  Value=3.6
  Product3 : Product
  V_km/h : Outport
  wires:
  Constant18/1 -> Product3/1
  Product3/1 -> V_km/h/1
  v/1 -> Product3/2

== system SimulinkProject/Subsystem1/m//s to km//h4 ==
  v : Inport
  Constant18 : Constant  Value=3.6
  Product3 : Product
  V_km/h : Outport
  wires:
  Constant18/1 -> Product3/1
  Product3/1 -> V_km/h/1
  v/1 -> Product3/2

== system SimulinkProject/Subsystem1/m//s to km//h5 ==
  v : Inport
  Constant18 : Constant  Value=3.6
  Product3 : Product
  V_km/h : Outport
  wires:
  Constant18/1 -> Product3/1
  Product3/1 -> V_km/h/1
  v/1 -> Product3/2

== matlab function SimulinkProject/Kalman ==
  data: a_acc input; v_est output; v_air input; valid input
function v_est = kalman_partial(a_acc, v_air, valid)
%#codegen

dt = 1/3200;     % set to your sample time
Q  = 1;         % tune
R  = 20;        % tune

persistent v P
if isempty(v)
    v = v_air;
    P = 100;
end

% Prediction from accelerometer
v_pred = v + a_acc * dt;
P_pred = P + Q;

if valid > 0.5
    % Correction only when airspeed is reliable
    K = P_pred / (P_pred + R);
    v = v_pred + K * (v_air - v_pred);
    P = (1 - K) * P_pred;
else
    % No airspeed correction
    v = v_pred;
    P = P_pred;
end

v_est = v;

== matlab function SimulinkProject/Kalman-Filter/test ==
  data: a_acc input; v_acc input; v_est output; v_air input; h_baro input; gamma input; valid input; v_init input; dv_baro output; dv_baro_sum output
function [v_est, dv_baro, dv_baro_sum] = kalman_3sensor(a_acc, v_acc, v_air, h_baro, gamma, valid, v_init)
%#codegen

dt = 1/3200;

Qv = 5.0;
Qh = 0.1;
Qb = 0.001;

R_air_valid   = 1.0;
R_air_invalid = 50000;
R_accv        = 2.0;
R_h           = 0.0001;

persistent x P dv_sum
if isempty(x)
    x = [v_init; h_baro; 0];   % [v; h; acc_bias]
    P = diag([100, 10, 1]);
    dv_sum = 0;
end

v = x(1);
h = x(2);
b = x(3);

% Prediction
v_pred = v + (a_acc - b)*dt;
h_pred = h + v*sin(gamma)*dt;
b_pred = b;

x_pred = [v_pred; h_pred; b_pred];

F = [1, 0, -dt;
     sin(gamma)*dt, 1, 0;
     0, 0, 1];

Q = diag([Qv, Qh, Qb]);

x = x_pred;
P = F*P*F' + Q;

% Integrated acceleration speed update
H_accv = [1 0 0];
K = P*H_accv'/(H_accv*P*H_accv' + R_accv);
x = x + K*(v_acc - H_accv*x);
P = (eye(3)-K*H_accv)*P;

% Airspeed update: strong if valid, almost ignored if invalid
H_air = [1 0 0];

if valid > 0.5
    R_air_now = R_air_valid;
else
    R_air_now = R_air_invalid;
end

K = P*H_air'/(H_air*P*H_air' + R_air_now);
x = x + K*(v_air - H_air*x);
P = (eye(3)-K*H_air)*P;

% Barometer update
x_before_baro = x;

H_h = [0 1 0];
K = P*H_h'/(H_h*P*H_h' + R_h);
x = x + K*(h_baro - H_h*x);
P = (eye(3)-K*H_h)*P;

% Outputs
v_est = x(1);

dv_baro = x(1) - x_before_baro(1);
dv_sum = dv_sum + dv_baro;
dv_baro_sum = dv_sum;

== matlab function SimulinkProject/MATLAB Function1 ==
  data: a_acc input; v_est output; v_air input; valid input
function v_est = kalman_speed_bias(a_acc, v_air, valid)
%#codegen

dt = 1/3200;   % change to your sample time

Qv = 0.5;       % speed uncertainty
Qb = 0.01;    % airspeed bias can slowly change
R  = 400;      % airspeed noise

persistent x P
if isempty(x)
    x = [13; 0];      % [speed; airspeed_bias]
    P = diag([100, 100]);
end

% Prediction
A = [1 0;
     0 1];

B = [dt;
     0];

Q = diag([Qv Qb]);

x_pred = A*x + B*a_acc;
P_pred = A*P*A' + Q;

% Measurement: v_air = speed + bias
H = [1 1];

if valid > 0.5
    K = P_pred*H'/(H*P_pred*H' + R);
    x = x_pred + K*(v_air - H*x_pred);
    P = (eye(2) - K*H)*P_pred;
else
    x = x_pred;
    P = P_pred;
end

v_est = x(1);

== matlab function SimulinkProject/MATLAB Function2 ==
  data: a_acc input; v_est output; v_air input; h_baro input; gamma input; valid input
function v_est = kalman_3sensor(a_acc, v_air, h_baro, gamma, valid)
%#codegen

dt = 1/3200;

Qv = 0.5;
Qh = 0.1;
Qb = 0.001;

R_air = 10000;
R_h   = 0.25;     % baro noise variance, e.g. 0.5m RMS -> 0.25

persistent x P
if isempty(x)
    x = [v_air; h_baro; 0];   % [speed; height; acc_bias]
    P = diag([100, 10, 1]);
end

v = x(1);
h = x(2);
b = x(3);

% Prediction
v_pred = v + (a_acc - b)*dt;
h_pred = h + v*sin(gamma)*dt;
b_pred = b;

x_pred = [v_pred; h_pred; b_pred];

P_pred = P + diag([Qv Qh Qb]);

x = x_pred;
P = P_pred;

% Airspeed update only in good zone
if valid > 0.5
    H_air = [1 0 0];
    K = P*H_air'/(H_air*P*H_air' + R_air);
    x = x + K*(v_air - H_air*x);
    P = (eye(3)-K*H_air)*P;
end

% Barometer height update
H_h = [0 1 0];
K = P*H_h'/(H_h*P*H_h' + R_h);
x = x + K*(h_baro - H_h*x);
P = (eye(3)-K*H_h)*P;

v_est = x(1);

== matlab function SimulinkProject/BEST ==
  data: a_acc input; v_est output; v_air input; h_baro input; gamma input; valid input; v_init input
function v_est = kalman_3sensor(a_acc, v_air, h_baro, gamma, valid, v_init)
%#codegen

dt = 1/3200;

Qv = 0.5;
Qh = 0.1;
Qb = 0.01;

R_air = 50000;
R_h   = 0.25;     % baro noise variance, e.g. 0.5m RMS -> 0.25

persistent x P
if isempty(x)
    x = [v_init; h_baro; 0];   % [speed; height; acc_bias]
    P = diag([100, 10, 1]);
end

v = x(1);
h = x(2);
b = x(3);

% Prediction
v_pred = v + (a_acc - b)*dt;
h_pred = h + v*sin(gamma)*dt;
b_pred = b;

x_pred = [v_pred; h_pred; b_pred];

P_pred = P + diag([Qv Qh Qb]);

x = x_pred;
P = P_pred;

% Airspeed update only in good zone
if valid > 0.5
    H_air = [1 0 0];
    K = P*H_air'/(H_air*P*H_air' + R_air);
    x = x + K*(v_air - H_air*x);
    P = (eye(3)-K*H_air)*P;
end

% Barometer height update
H_h = [0 1 0];
K = P*H_h'/(H_h*P*H_h' + R_h);
x = x + K*(h_baro - H_h*x);
P = (eye(3)-K*H_h)*P;

v_est = x(1);

== matlab function SimulinkProject/BEST1 ==
  data: a_acc input; v_est output; v_air input; h_baro input; gamma input; valid input; v_init input
function v_est = kalman_3sensor(a_acc, v_air, h_baro, gamma, valid, v_init)
%#codegen

dt = 1/3200;

Qv = 0.5;
Qh = 0.1;
Qb = 0.01;

R_air = 50000;
R_h   = 0.25;     % baro noise variance, e.g. 0.5m RMS -> 0.25

persistent x P
if isempty(x)
    x = [v_init; h_baro; 0];   % [speed; height; acc_bias]
    P = diag([100, 10, 1]);
end

v = x(1);
h = x(2);
b = x(3);

% Prediction
v_pred = v + (a_acc - b)*dt;
h_pred = h + v*sin(gamma)*dt;
b_pred = b;

x_pred = [v_pred; h_pred; b_pred];

P_pred = P + diag([Qv Qh Qb]);

x = x_pred;
P = P_pred;

% Airspeed update only in good zone
if valid > 0.5
    H_air = [1 0 0];
    K = P*H_air'/(H_air*P*H_air' + R_air);
    x = x + K*(v_air - H_air*x);
    P = (eye(3)-K*H_air)*P;
end

% Barometer height update
H_h = [0 1 0];
K = P*H_h'/(H_h*P*H_h' + R_h);
x = x + K*(h_baro - H_h*x);
P = (eye(3)-K*H_h)*P;

v_est = x(1);

== matlab function SimulinkProject/test1 ==
  data: a_acc input; v_acc input; v_est output; v_air input; h_baro input; gamma input; valid input; v_init input; dv_baro output; dv_baro_sum output
function [v_est, dv_baro, dv_baro_sum] = kalman_3sensor(a_acc, v_acc, v_air, h_baro, gamma, valid, v_init)
%#codegen

dt = 1/3200;

Qv = 8.0;
Qh = 0.1;
Qb = 0.001;

R_air_valid   = 1.0;
R_air_invalid = 50000;
R_accv        = 5.0;
R_h           = 0.0001;

persistent x P dv_sum
if isempty(x)
    x = [v_init; h_baro; 0];
    P = diag([100, 10, 1]);
    dv_sum = 0;
end

v = x(1);
h = x(2);
b = x(3);

% Prediction
v_pred = v + (a_acc - b)*dt;
h_pred = h + v*sin(gamma)*dt;
b_pred = b;

x_pred = [v_pred; h_pred; b_pred];

F = [1, 0, -dt;
     sin(gamma)*dt, 1, 0;
     0, 0, 1];

Q = diag([Qv, Qh, Qb]);
P_pred = F*P*F' + Q;

x = x_pred;
P = P_pred;

% Integrated acceleration speed update
H_accv = [1 0 0];
K = P*H_accv'/(H_accv*P*H_accv' + R_accv);
x = x + K*(v_acc - H_accv*x);
P = (eye(3)-K*H_accv)*P;

% Airspeed update: strong if valid, weak if invalid
H_air = [1 0 0];

if valid > 0.5
    R_air_now = R_air_valid;
else
    R_air_now = R_air_invalid;
end

K = P*H_air'/(H_air*P*H_air' + R_air_now);
x = x + K*(v_air - H_air*x);
P = (eye(3)-K*H_air)*P;

% Barometer height update
x_before_baro = x;

H_h = [0 1 0];
K = P*H_h'/(H_h*P*H_h' + R_h);
x = x + K*(h_baro - H_h*x);
P = (eye(3)-K*H_h)*P;

v_est = x(1);

dv_baro = x(1) - x_before_baro(1);
dv_sum = dv_sum + dv_baro;
dv_baro_sum = dv_sum;
